simulink model "plant_control_inner"  (R2023a)
settings: Solver=FixedStepAuto  StartTime=0.0  StopTime=10.0  FixedStep=0.01  RelTol=1e-3
values from neighbouring files (symbols this model uses):
  g = 9.81    [full_loop.m]    (also in inner_loop.m)
  KI = K(:,1:2)    [LQR_PI.m]    (also in full_loop.m = K(:,1:nref); inner_loop.m = K(:,1:3))
  Kp_x = K(:,3:5)    [LQR_PI.m]    (also in full_loop.m = K(:,nref+1:np+nref); inner_loop.m = K(:,4:9))
  Kp_xref = K(:,6:7)    [LQR_PI.m]    (also in full_loop.m = K(:,np+nref+1:end); inner_loop.m = K(:,10:12))
  m = 10    [full_loop.m]    (also in inner_loop.m)
  sys_p = ss(Ap, Bp, Cp, Dp)    [LQR_PI.m]    (also in full_loop.m = ss(Ap, Bp, Cp([1:3,9],:), zeros(nref, mp)); inner_loop.m = ss(Ap(1:np, 1:np), Bp(1:np, :), Cp(:, 1:np), Dp))
  sys_ref = ss(A_ref, B_ref, C_ref, D_ref)    [LQR_PI.m]    (also in full_loop.m; inner_loop.m)
libraries: simulink_extras x3, shared6dof x1
settings Model: Creator=timme  LastModifiedBy=timme
settings OptimizationCC: BlockReduction=off  DefaultParameterBehavior=Inlined  BufferReuse=off

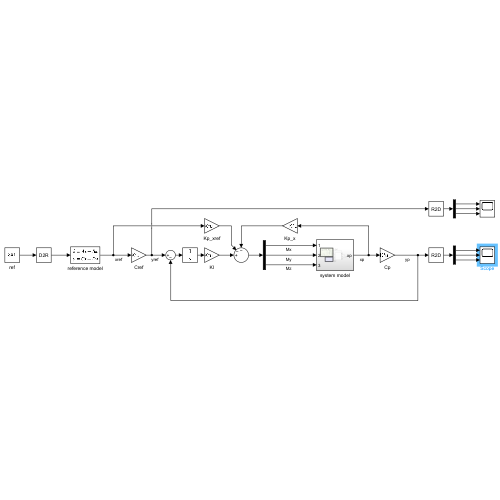
[thumbnail: Simulink's stored preview of the top-level diagram]
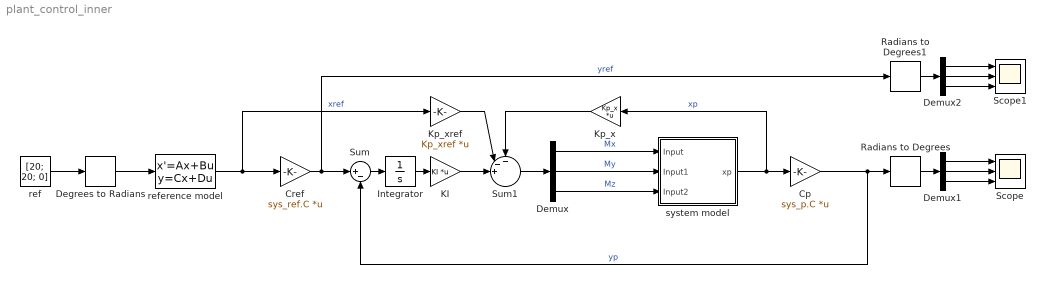
== system plant_control_inner ==
  Cp : Gain  Gain=sys_p.C  Multiplication=Matrix(K*u)
  Cref : Gain  Gain=sys_ref.C  Multiplication=Matrix(K*u)
  Degrees to Radians : simulink_extras/Transformations/Degrees to Radians
  Demux : Demux  Outputs=3
  Demux1 : Demux  Outputs=3
  Demux2 : Demux  Outputs=3
  Integrator : Integrator
  KI : Gain  Gain=KI  Multiplication=Matrix(K*u)
  Kp_x : Gain  Gain=Kp_x  Multiplication=Matrix(K*u)
  Kp_xref : Gain  Gain=Kp_xref  Multiplication=Matrix(K*u)
  Radians to Degrees : simulink_extras/Transformations/Radians to Degrees
  Radians to Degrees1 : simulink_extras/Transformations/Radians to Degrees
  Scope : Scope  NumInputPorts=3
  Scope1 : Scope  NumInputPorts=3
  Sum : Sum  Inputs=|+-
  Sum1 : Sum  Inputs=--+||
  ref : Constant  Value=[20; 20; 0]
  reference model : StateSpace  A=sys_ref.A  B=sys_ref.B  C=sys_ref.C  D=sys_ref.D  InitialCondition=0
  system model : Subsystem
  wires:
  Demux/1 -> system model/1(Input)  "Mx"
  Demux/2 -> system model/2(Input1)  "My"
  Demux/3 -> system model/3(Input2)  "Mz"
  system model/1(xp) -> Kp_x/1, Cp/1  "xp"
  ref/1 -> Degrees to Radians/1
  reference model/1 -> Kp_xref/1, Cref/1  "xref"
  Cref/1 -> Radians to Degrees1/1, Sum/1  "yref"
  Sum/1 -> Integrator/1
  Cp/1 -> Radians to Degrees/1, Sum/2  "yp"
  Integrator/1 -> KI/1
  KI/1 -> Sum1/3
  Kp_xref/1 -> Sum1/2
  Kp_x/1 -> Sum1/1
  Sum1/1 -> Demux/1
  Degrees to Radians/1 -> reference model/1
  Demux1/1 -> Scope/1
  Demux1/2 -> Scope/2
  Demux1/3 -> Scope/3
  Radians to Degrees/1 -> Demux1/1
  Demux2/1 -> Scope1/1
  Demux2/2 -> Scope1/2
  Radians to Degrees1/1 -> Demux2/1
  Demux2/3 -> Scope1/3

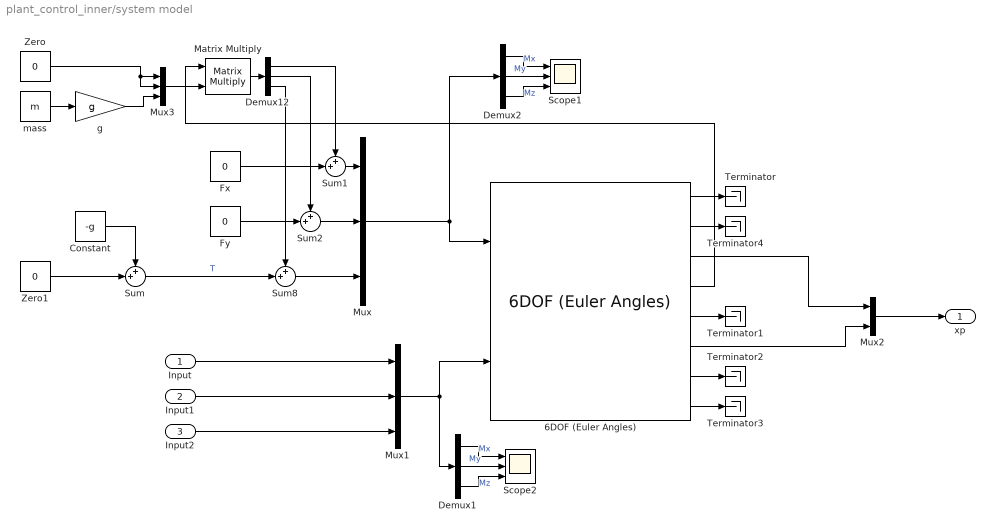
== system plant_control_inner/system model ==
  Input : Inport
  Input1 : Inport  Port=2
  Input2 : Inport  Port=3
  6DOF (Euler Angles) : shared6dof/6DOF (Euler Angles)  units=Metric (MKS)  mtype=Fixed  rep=Euler Angles  xme_0=[0 0 0]  Vm_0=[0 0 0]  eul_0=[0 0 0]  pm_0=[0 0 0]  mass_0=m  mass_e=0.5  mass_f=2.0  inertia=I  inertia_e=eye(3)  inertia_f=2*eye(3)  k_quat=1.0  vre_flag=on  abi_flag=off  aMode=0  xme_statename=''  Vm_statename=''  eul_statename=''  quat_statename=''  pm_statename=''  mass_statename=''
  Constant : Constant  Value=-g
  Demux1 : Demux  Outputs=3
  Demux12 : Demux  Outputs=3
  Demux2 : Demux  Outputs=3
  Fx : Constant  Value=0
  Fy : Constant  Value=0
  Matrix Multiply : Product  Inputs=**  Multiplication=Matrix(*)
  Mux : Mux  Inputs=3
  Mux1 : Mux  Inputs=3
  Mux2 : Mux  Inputs=2
  Mux3 : Mux  Inputs=3
  Scope1 : Scope  NumInputPorts=3
  Scope2 : Scope  NumInputPorts=3
  Sum{,1..2,8} (4 alike) : Sum  Inputs=++|
  Terminator{,1..4} (5 alike) : Terminator
  Zero : Constant  Value=0  OutDataTypeStr=Inherit: Inherit via back propagation
  Zero1 : Constant  Value=0  OutDataTypeStr=Inherit: Inherit via back propagation
  g : Gain  Gain=g
  mass : Constant  Value=m
  xp : Outport
  wires:
  Mux2/1 -> xp/1
  g/1 -> Mux3/3
  Demux1/2 -> Scope2/2  "My"
  Constant/1 -> Sum/1
  6DOF (Euler Angles)/6 -> Mux2/2
  Demux1/1 -> Scope2/1  "Mx"
  6DOF (Euler Angles)/3 -> Mux2/1
  Input/1 -> Mux1/1
  6DOF (Euler Angles)/4 -> Matrix Multiply/1
  Zero/1 -> Mux3/1, Mux3/2
  Demux2/1 -> Scope1/1  "Mx"
  Sum1/1 -> Mux/1
  Fx/1 -> Sum1/2
  Demux1/3 -> Scope2/3  "Mz"
  Sum8/1 -> Mux/3
  Sum/1 -> Sum8/2  "T"
  Zero1/1 -> Sum/2
  Fy/1 -> Sum2/2
  6DOF (Euler Angles)/5 -> Terminator1/1
  Demux12/3 -> Sum8/1
  6DOF (Euler Angles)/7 -> Terminator2/1
  Sum2/1 -> Mux/2
  Mux/1 -> Demux2/1, 6DOF (Euler Angles)/1
  Demux2/2 -> Scope1/2  "My"
  Input2/1 -> Mux1/3
  6DOF (Euler Angles)/2 -> Terminator4/1
  mass/1 -> g/1
  Input1/1 -> Mux1/2
  Mux1/1 -> 6DOF (Euler Angles)/2, Demux1/1
  Demux12/2 -> Sum2/1
  Demux12/1 -> Sum1/1
  6DOF (Euler Angles)/1 -> Terminator/1
  Demux2/3 -> Scope1/3  "Mz"
  Mux3/1 -> Matrix Multiply/2
  Matrix Multiply/1 -> Demux12/1
  6DOF (Euler Angles)/8 -> Terminator3/1
